simulink model "six"  (R2016b)
settings: Solver=ode4  StartTime=0.0  StopTime=10  FixedStep=0.001  RelTol=1e-3
values from neighbouring files (symbols this model uses):
  g = 9.8    [initialization.m]
  Jx = 0.007    [initialization.m]
  Jy = 0.184    [initialization.m]
  Jz = 0.184    [initialization.m]
  ksi_a = 0.6    [initialization.m]
  ksi_g = 0.7    [initialization.m]
  L = 0.9    [initialization.m]
  m = 4.81    [initialization.m]
  psiv0 = 0    [initialization.m]
  S = 0.0133    [initialization.m]
  Somega = 6*naturefrequency    [initialization.m]
  T = 1/a34    (= 0.0335307174903)    [initialization.m]
  Ta = 0.0059    [initialization.m]
  Tg = 0.006    [initialization.m]
  V0 = 1000    [initialization.m]
  xm0 = 0    [initialization.m]
  ym0 = 0    [initialization.m]
  zm0 = 0    [initialization.m]
libraries: aerolibatmos2 x1, simulink x1
settings Model: Creator=WangXuanLing  LastModifiedBy=asus
settings DataIOCC: LimitDataPoints=on  SaveFormat=Array
settings OptimizationCC: BlockReduction=off  BooleanDataType=off  LifeSpan=inf
settings DebuggingCC: SaveWithParameterizedLinksMsg=none  UnderspecifiedInitializationDetection=Classic  MergeDetectMultiDrivingBlocksExec=none  SignalResolutionControl=TryResolveAllWithWarning  SFUnexpectedBacktrackingDiag=warning  SFNoUnconditionalDefaultTransitionDiag=warning  SFExecutionAtInitializationDiag=none
settings HardwareCC: ProdBitPerPointer=32  ProdBitPerSizeT=32  ProdBitPerPtrDiffT=32  ProdLargestAtomicFloat=None  ProdIntDivRoundTo=Undefined  ProdEndianess=Unspecified  ProdWordSize=32  ProdHWDeviceType=32-bit Generic  TargetUnknown=on
settings ModelReferenceCC: PropagateSignalLabelsOutOfModel=off
settings GRTTargetCC: TargetLangStandard=C89/C90 (ANSI)  GeneratePreprocessorConditionals=Disable all
settings ConfigComp: CovMetricSettings=dw  CovHtmlReporting=on  CovSaveCumulativeToWorkspaceVar=on  CovSaveSingleToWorkspaceVar=on  CovExternalEMLEnable=off  CovSFcnEnable=off

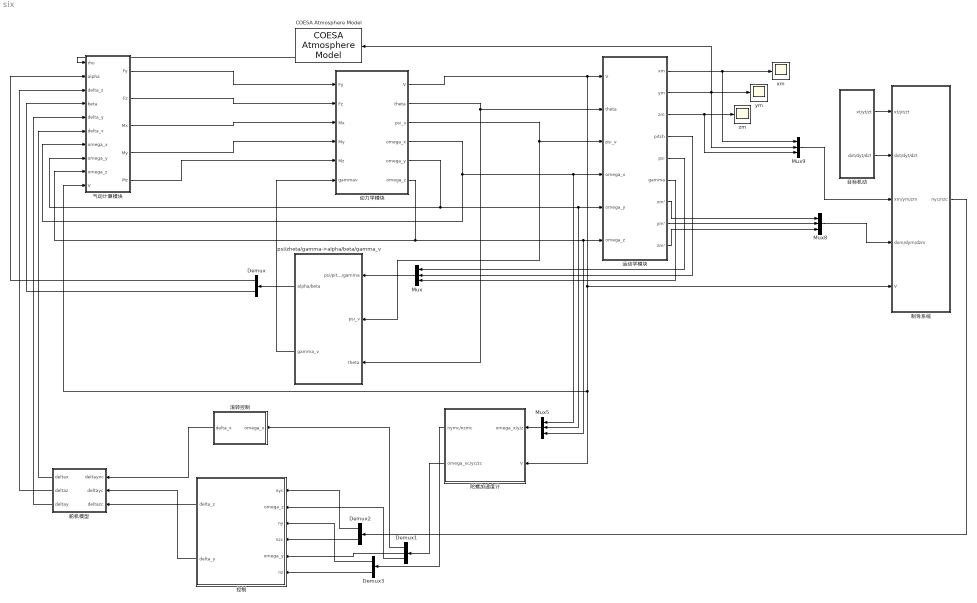
== system six ==
  COESA Atmosphere Model : aerolibatmos2/COESA Atmosphere Model  units=Metric (MKS)  spec=1976 COESA-extended U.S. Standard Atmosphere  model=Profile  profile_var=High temperature  profile_percent=1%  profile_alt=5 km (16404 ft)  envelope_var=High temperature  envelope_percent=1%  action=Warning
  Demux : Demux  Outputs=2
  Demux1 : Demux  Outputs=3
  Demux2 : Demux  Outputs=2
  Demux3 : Demux  Outputs=2
  Mux{,5,8..9} (4 alike) : Mux  Inputs=3
  psi/zheta/gamma->alpha/beta/gamma_v : Subsystem
  xm : Scope
  ym : Scope
  zm : Scope
  制导系统 : Subsystem
  动力学模块 : Subsystem
  控制 : Subsystem
  气动计算模块 : Subsystem
  滚转控制 : Subsystem
  目标机动 : Subsystem
  舵机模型 : Subsystem
  运动学模块 : Subsystem
  陀螺加速度计 : Subsystem
  wires:
  气动计算模块/1(Fy) -> 动力学模块/1(Fy)
  气动计算模块/2(Fz) -> 动力学模块/2(Fz)
  气动计算模块/3(Mx) -> 动力学模块/3(Mx)
  气动计算模块/4(My) -> 动力学模块/4(My)
  气动计算模块/5(Mz) -> 动力学模块/5(Mz)
  psi/zheta/gamma->alpha/beta/gamma_v/2(gamma_v) -> 动力学模块/6("gammav ")
  动力学模块/2(theta) -> psi/zheta/gamma->alpha/beta/gamma_v/3(theta), 运动学模块/2(theta)
  动力学模块/5(omega_y) -> 气动计算模块/8(omega_y), Mux5/2, 运动学模块/5(omega_y)
  动力学模块/6(omega_z) -> 气动计算模块/9(omega_z), Mux5/3, 运动学模块/6(omega_z)
  动力学模块/3(psi_v) -> psi/zheta/gamma->alpha/beta/gamma_v/2(psi_v), 运动学模块/3(psi_v)
  Demux/2 -> 气动计算模块/4(beta)
  Demux/1 -> 气动计算模块/2(alpha)
  运动学模块/5(psi) -> Mux/1
  运动学模块/4(pitch) -> Mux/2
  运动学模块/7(xm') -> Mux8/1
  运动学模块/8(ym') -> Mux8/2
  运动学模块/9(zm') -> Mux8/3
  动力学模块/1(V) -> 陀螺加速度计/2(V), 气动计算模块/10(V), 制导系统/5(V), 运动学模块/1(V)
  运动学模块/2(ym) -> COESA Atmosphere Model/1, ym/1, Mux9/2
  动力学模块/4(omega_x) -> 气动计算模块/7(omega_x), Mux5/1, 运动学模块/4(omega_x)
  滚转控制/1(delta_x) -> 舵机模型/1(deltayxc)
  控制/1(delta_z) -> 舵机模型/3(deltazc)
  控制/2(delta_y) -> 舵机模型/2(deltayc)
  运动学模块/6(gamma) -> Mux/3
  运动学模块/3(zm) -> zm/1, Mux9/3
  运动学模块/1(xm) -> Mux9/1, xm/1
  舵机模型/1(deltax) -> 气动计算模块/6(delta_x)
  舵机模型/2(deltaz) -> 气动计算模块/3(delta_z)
  舵机模型/3(deltay) -> 气动计算模块/5(delta_y)
  psi/zheta/gamma->alpha/beta/gamma_v/1(alpha/beta) -> Demux/1
  Mux/1 -> psi/zheta/gamma->alpha/beta/gamma_v/1(psi/pitch/gamma)
  制导系统/1(nyc/nzc) -> Demux2/1
  目标机动/2(dxt/dyt/dzt) -> 制导系统/2(dxt/dyt/dzt)
  目标机动/1(xt/yt/zt) -> 制导系统/1(xt/yt/zt)
  Mux8/1 -> 制导系统/4(dxm/dym/dzm)
  Mux9/1 -> 制导系统/3(xm/ym/zm)
  陀螺加速度计/2(omega_xc/yc/zc) -> Demux1/1
  陀螺加速度计/1(nymc/nzmc) -> Demux3/1
  Mux5/1 -> 陀螺加速度计/1(omega_x/y/z)
  COESA Atmosphere Model/4 -> 气动计算模块/1(rho)
  Demux1/1 -> 滚转控制/1(omega_x)
  Demux1/2 -> 控制/5(omega_y)
  Demux1/3 -> 控制/2(omega_z)
  Demux2/1 -> 控制/1(nyc)
  Demux2/2 -> 控制/4(nzc)
  Demux3/1 -> 控制/3(ny)
  Demux3/2 -> 控制/6(nz)

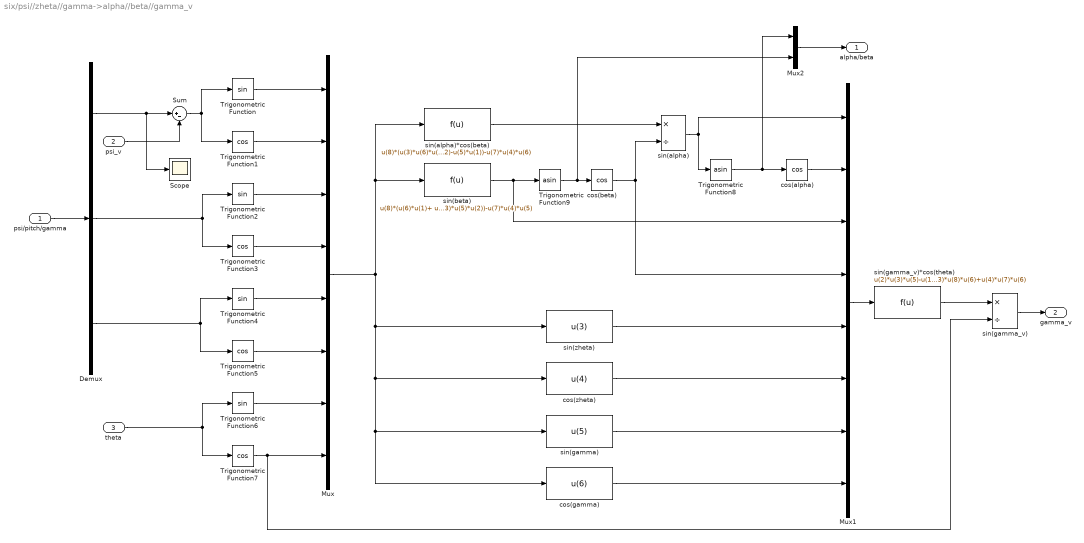
== system six/psi//zheta//gamma->alpha//beta//gamma_v ==
  psi/pitch/gamma : Inport
  psi_v : Inport  Port=2
  theta : Inport  Port=3
  Demux : Demux  Outputs=3
  Mux : Mux  Inputs=8
  Mux1 : Mux  Inputs=8
  Mux2 : Mux  Inputs=2
  Scope : Scope
  Sum : Sum  Inputs=|+-
  Trigonometric Function{,2,4,6} (4 alike) : Trigonometry
  Trigonometric Function{1,3,5,7} (4 alike) : Trigonometry  Operator=cos
  Trigonometric Function8 : Trigonometry  Operator=asin
  Trigonometric Function9 : Trigonometry  Operator=asin
  cos(alpha) : Trigonometry  Operator=cos
  cos(beta) : Trigonometry  Operator=cos
  cos(gamma) : Fcn  Expr=u(6)
  cos(zheta) : Fcn  Expr=u(4)
  sin(alpha) : Product  Inputs=*/
  sin(alpha)*cos(beta) : Fcn  Expr=u(8)*(u(3)*u(6)*u(2)-u(5)*u(1))-u(7)*u(4)*u(6)
  sin(beta) : Fcn  Expr=u(8)*(u(6)*u(1)+ u(3)*u(5)*u(2))-u(7)*u(4)*u(5)
  sin(gamma) : Fcn  Expr=u(5)
  sin(gamma_v) : Product  Inputs=*/
  sin(gamma_v)*cos(theta) : Fcn  Expr=u(2)*u(3)*u(5)-u(1)*u(3)*u(8)*u(6)+u(4)*u(7)*u(6)
  sin(zheta) : Fcn  Expr=u(3)
  alpha/beta : Outport
  gamma_v : Outport  Port=2
  wires:
  psi/pitch/gamma/1 -> Demux/1
  Demux/1 -> Scope/1, Sum/1
  Sum/1 -> Trigonometric Function/1, Trigonometric Function1/1
  Demux/2 -> Trigonometric Function3/1, Trigonometric Function2/1
  Demux/3 -> Trigonometric Function4/1, Trigonometric Function5/1
  Trigonometric Function/1 -> Mux/1
  Trigonometric Function1/1 -> Mux/2
  Trigonometric Function2/1 -> Mux/3
  Trigonometric Function3/1 -> Mux/4
  Trigonometric Function4/1 -> Mux/5
  Trigonometric Function5/1 -> Mux/6
  theta/1 -> Trigonometric Function7/1, Trigonometric Function6/1
  Trigonometric Function6/1 -> Mux/7
  Trigonometric Function7/1 -> Mux/8, sin(gamma_v)/2
  sin(beta)/1 -> Mux1/3, Trigonometric Function9/1
  Trigonometric Function9/1 -> Mux2/2, cos(beta)/1
  sin(alpha)*cos(beta)/1 -> sin(alpha)/1
  cos(beta)/1 -> Mux1/4, sin(alpha)/2
  sin(alpha)/1 -> Mux1/1, Trigonometric Function8/1
  Trigonometric Function8/1 -> Mux2/1, cos(alpha)/1
  cos(alpha)/1 -> Mux1/2
  sin(zheta)/1 -> Mux1/5
  cos(zheta)/1 -> Mux1/6
  sin(gamma)/1 -> Mux1/7
  cos(gamma)/1 -> Mux1/8
  sin(gamma_v)*cos(theta)/1 -> sin(gamma_v)/1
  sin(gamma_v)/1 -> gamma_v/1
  psi_v/1 -> Sum/2
  Mux/1 -> cos(gamma)/1, sin(gamma)/1, cos(zheta)/1, sin(zheta)/1, sin(alpha)*cos(beta)/1, sin(beta)/1
  Mux1/1 -> sin(gamma_v)*cos(theta)/1
  Mux2/1 -> alpha/beta/1

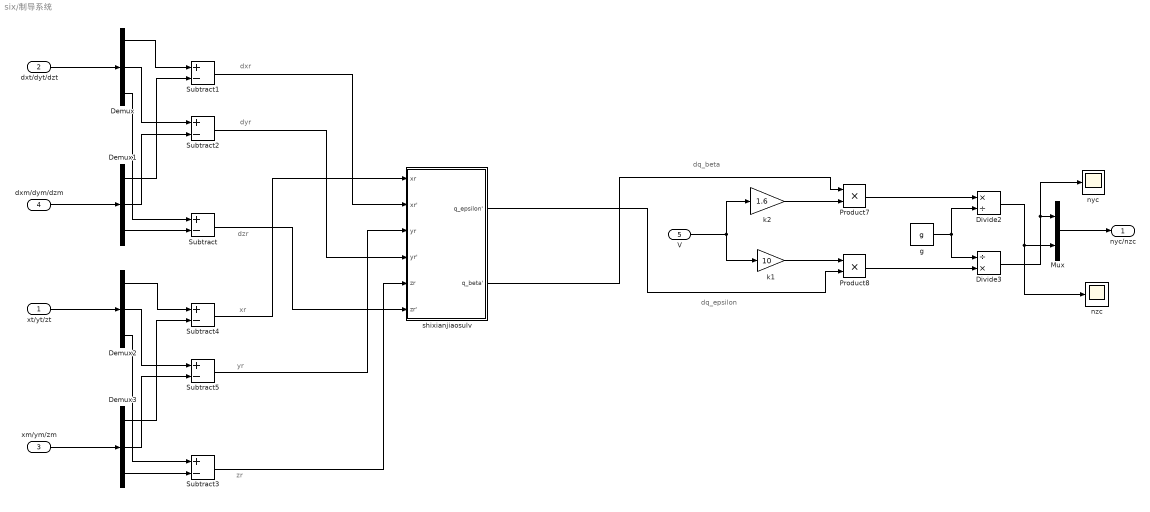
== system six/制导系统 ==
  note: dq_epsilon
  note: zr
  note: yr
  note: xr
  note: dzr
  note: dyr
  note: dxr
  note: dq_beta
  xt/yt/zt : Inport
  dxt/dyt/dzt : Inport  Port=2
  xm/ym/zm : Inport  Port=3
  dxm/dym/dzm : Inport  Port=4
  V : Inport  Port=5
  Demux{,1..3} (4 alike) : Demux  Outputs=3
  Divide2 : Product  Inputs=*/
  Divide3 : Product  Inputs=/*
  Mux : Mux  Inputs=2
  Product7 : Product
  Product8 : Product
  Subtract{,1..5} (6 alike) : Sum  Inputs=+-
  g : Constant  Value=g
  k1 : Gain  Gain=10
  k2 : Gain  Gain=1.6
  nyc : Scope
  nzc : Scope
  shixianjiaosulv : Subsystem
  nyc/nzc : Outport
  wires:
  Demux/3 -> Subtract/1
  Demux/2 -> Subtract2/1
  dxm/dym/dzm/1 -> Demux1/1
  dxt/dyt/dzt/1 -> Demux/1
  k2/1 -> Product7/2
  Subtract5/1 -> shixianjiaosulv/3(yr)
  Product7/1 -> Divide2/1
  g/1 -> Divide3/1, Divide2/2
  Demux3/3 -> Subtract3/2
  Mux/1 -> nyc/nzc/1
  Demux1/3 -> Subtract/2
  Demux2/1 -> Subtract4/1
  V/1 -> k1/1, k2/1
  Demux3/1 -> Subtract4/2
  Product8/1 -> Divide3/2
  Demux2/2 -> Subtract5/1
  xm/ym/zm/1 -> Demux3/1
  xt/yt/zt/1 -> Demux2/1
  Subtract3/1 -> shixianjiaosulv/5(zr)
  k1/1 -> Product8/1
  Demux3/2 -> Subtract5/2
  Demux2/3 -> Subtract3/1
  Demux1/1 -> Subtract1/2
  Demux/1 -> Subtract1/1
  Demux1/2 -> Subtract2/2
  Divide2/1 -> nzc/1, Mux/2
  Divide3/1 -> Mux/1, nyc/1
  shixianjiaosulv/1(q_epsilon') -> Product8/2
  shixianjiaosulv/2(q_beta') -> Product7/1
  Subtract4/1 -> shixianjiaosulv/1(xr)
  Subtract1/1 -> shixianjiaosulv/2(xr')
  Subtract2/1 -> shixianjiaosulv/4(yr')
  Subtract/1 -> shixianjiaosulv/6(zr')

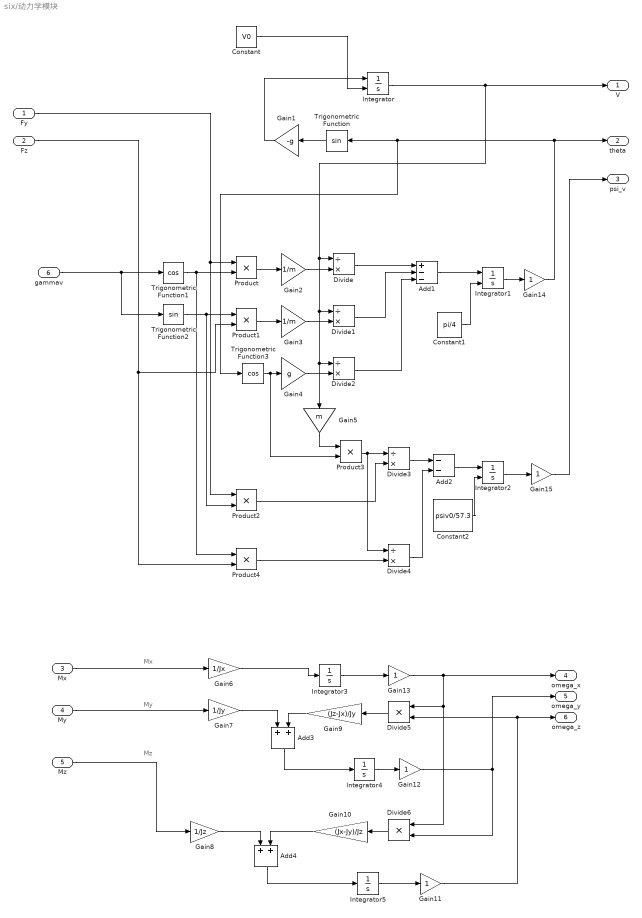
== system six/动力学模块 ==
  note: Mz
  note: My
  note: Mx
  Fy : Inport
  Fz : Inport  Port=2
  Mx : Inport  Port=3
  My : Inport  Port=4
  Mz : Inport  Port=5
  "gammav " : Inport  Port=6
  Add1 : Sum  Inputs=+--
  Add2 : Sum  Inputs=--
  Add3 : Sum
  Add4 : Sum
  Constant : Constant  Value=V0
  Constant1 : Constant  Value=pi/4
  Constant2 : Constant  Value=psiv0/57.3
  Divide{,1..4} (5 alike) : Product  Inputs=/*
  Divide5 : Product  Inputs=**
  Divide6 : Product  Inputs=**
  Gain1 : Gain  Gain=-g
  Gain10 : Gain  Gain=(Jx-Jy)/Jz
  Gain{11..15} (5 alike) : Gain
  Gain2 : Gain  Gain=1/m
  Gain3 : Gain  Gain=1/m
  Gain4 : Gain  Gain=g
  Gain5 : Gain  Gain=m
  Gain6 : Gain  Gain=1/Jx
  Gain7 : Gain  Gain=1/Jy
  Gain8 : Gain  Gain=1/Jz
  Gain9 : Gain  Gain=(Jz-Jx)/Jy
  Integrator : Integrator  InitialConditionSource=external
  Integrator1 : Integrator  InitialConditionSource=external
  Integrator2 : Integrator  InitialConditionSource=external
  Integrator3 : Integrator
  Integrator4 : Integrator
  Integrator5 : Integrator
  Product{,1..4} (5 alike) : Product
  Trigonometric Function : Trigonometry
  Trigonometric Function1 : Trigonometry  Operator=cos
  Trigonometric Function2 : Trigonometry
  Trigonometric Function3 : Trigonometry  Operator=cos
  V : Outport
  theta : Outport  Port=2
  psi_v : Outport  Port=3
  omega_x : Outport  Port=4
  omega_y : Outport  Port=5
  omega_z : Outport  Port=6
  wires:
  Fy/1 -> Product/1, Product2/1
  Fz/1 -> Product4/2, Product1/2
  Trigonometric Function/1 -> Gain1/1
  Gain1/1 -> Integrator/1
  "gammav "/1 -> Trigonometric Function2/1, Trigonometric Function1/1
  Trigonometric Function1/1 -> Product4/1, Product/2
  Product/1 -> Gain2/1
  Gain2/1 -> Divide/2
  Gain3/1 -> Divide1/2
  Product1/1 -> Gain3/1
  Divide/1 -> Add1/1
  Divide1/1 -> Add1/2
  Constant/1 -> Integrator/2
  Trigonometric Function3/1 -> Product3/2, Gain4/1
  Gain4/1 -> Divide2/2
  Divide2/1 -> Add1/3
  Add1/1 -> Integrator1/1
  Constant1/1 -> Integrator1/2
  Trigonometric Function2/1 -> Product1/1, Product2/2
  Gain5/1 -> Product3/1
  Product3/1 -> Divide4/1, Divide3/1
  Product2/1 -> Divide3/2
  Divide3/1 -> Add2/1
  Product4/1 -> Divide4/2
  Divide4/1 -> Add2/2
  Add2/1 -> Integrator2/1
  Constant2/1 -> Integrator2/2
  Mx/1 -> Gain6/1
  My/1 -> Gain7/1
  Mz/1 -> Gain8/1
  Gain6/1 -> Integrator3/1
  Integrator3/1 -> Gain13/1
  Gain7/1 -> Add3/1
  Divide5/1 -> Gain9/1
  Gain9/1 -> Add3/2
  Add3/1 -> Integrator4/1
  Gain8/1 -> Add4/1
  Gain12/1 -> omega_y/1, Divide6/2
  Divide6/1 -> Gain10/1
  Gain10/1 -> Add4/2
  Add4/1 -> Integrator5/1
  Gain11/1 -> Divide5/2, omega_z/1
  Integrator/1 -> V/1, Divide/1, Gain5/1, Divide2/1, Divide1/1
  Integrator1/1 -> Gain14/1
  Integrator2/1 -> Gain15/1
  Integrator5/1 -> Gain11/1
  Integrator4/1 -> Gain12/1
  Gain14/1 -> theta/1, Trigonometric Function/1, Trigonometric Function3/1
  Gain15/1 -> psi_v/1
  Gain13/1 -> omega_x/1, Divide6/1, Divide5/1

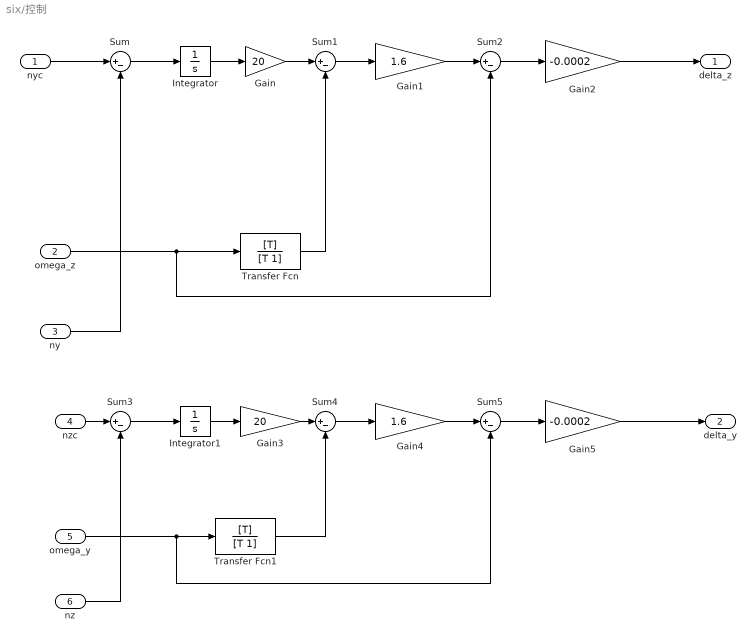
== system six/控制 ==
  nyc : Inport
  omega_z : Inport  Port=2
  ny : Inport  Port=3
  nzc : Inport  Port=4
  omega_y : Inport  Port=5
  nz : Inport  Port=6
  Gain : Gain  Gain=20
  Gain1 : Gain  Gain=1.6
  Gain2 : Gain  Gain=-0.0002
  Gain3 : Gain  Gain=20
  Gain4 : Gain  Gain=1.6
  Gain5 : Gain  Gain=-0.0002
  Integrator : Integrator
  Integrator1 : Integrator
  Sum{,1..5} (6 alike) : Sum  Inputs=|+-
  Transfer Fcn : TransferFcn  Numerator=[T]  Denominator=[T 1]
  Transfer Fcn1 : TransferFcn  Numerator=[T]  Denominator=[T 1]
  delta_z : Outport
  delta_y : Outport  Port=2
  wires:
  Sum3/1 -> Integrator1/1
  Integrator/1 -> Gain/1
  Sum4/1 -> Gain4/1
  Sum/1 -> Integrator/1
  Integrator1/1 -> Gain3/1
  Sum2/1 -> Gain2/1
  Gain4/1 -> Sum5/1
  Sum1/1 -> Gain1/1
  Gain1/1 -> Sum2/1
  Sum5/1 -> Gain5/1
  Gain3/1 -> Sum4/1
  Gain/1 -> Sum1/1
  Gain2/1 -> delta_z/1
  Gain5/1 -> delta_y/1
  omega_y/1 -> Sum5/2, Transfer Fcn1/1
  Transfer Fcn1/1 -> Sum4/2
  nyc/1 -> Sum/1
  ny/1 -> Sum/2
  omega_z/1 -> Sum2/2, Transfer Fcn/1
  Transfer Fcn/1 -> Sum1/2
  nz/1 -> Sum3/2
  nzc/1 -> Sum3/1

== system six/气动计算模块 ==
  rho : Inport
  alpha : Inport  Port=2
  delta_z : Inport  Port=3
  beta : Inport  Port=4
  delta_y : Inport  Port=5
  delta_x : Inport  Port=6
  omega_x : Inport  Port=7
  omega_y : Inport  Port=8
  omega_z : Inport  Port=9
  V : Inport  Port=10
  Gain : Gain  Gain=0.5
  Product : Product  Inputs=3
  qidongli : Subsystem
  qidongliju : Subsystem
  Fy : Outport
  Fz : Outport  Port=2
  Mx : Outport  Port=3
  My : Outport  Port=4
  Mz : Outport  Port=5
  wires:
  qidongli/2(Fz) -> Fz/1
  delta_x/1 -> qidongliju/1(delta_x)
  delta_y/1 -> qidongliju/4(delta_y), qidongli/5(delta_y)
  beta/1 -> qidongli/4(beta), qidongliju/6(beta)
  delta_z/1 -> qidongli/2(delta_z), qidongliju/7(delta_z)
  Gain/1 -> qidongli/3(q), qidongliju/3(q)
  alpha/1 -> qidongli/1(alpha), qidongliju/9(alpha)
  qidongliju/1(Mx) -> Mx/1
  qidongliju/2(My) -> My/1
  qidongli/1(Fy) -> Fy/1
  V/1 -> Product/1, Product/2
  Product/1 -> Gain/1
  rho/1 -> Product/3
  omega_x/1 -> qidongliju/2(omega_x)
  omega_y/1 -> qidongliju/5(omega_y)
  omega_z/1 -> qidongliju/8(omega_z)
  qidongliju/3(Mz) -> Mz/1

== system six/滚转控制 ==
  omega_x : Inport
  Integrator : Integrator
  Ka1 : Gain  Gain=70
  Ka2 : Gain  Gain=0
  Kb1 : Gain  Gain=-0.015
  Sine Wave : Sin  Amplitude=1/57.3  Frequency=10  SampleTime=0
  Sum2 : Sum  Inputs=|+-
  Sum3 : Sum  Inputs=|+-
  delta_x : Outport
  wires:
  Sine Wave/1 -> Ka2/1
  Sum2/1 -> Ka1/1
  Sum3/1 -> Kb1/1
  Kb1/1 -> delta_x/1
  omega_x/1 -> Integrator/1, Sum3/2
  Ka2/1 -> Sum2/1
  Ka1/1 -> Sum3/1
  Integrator/1 -> Sum2/2

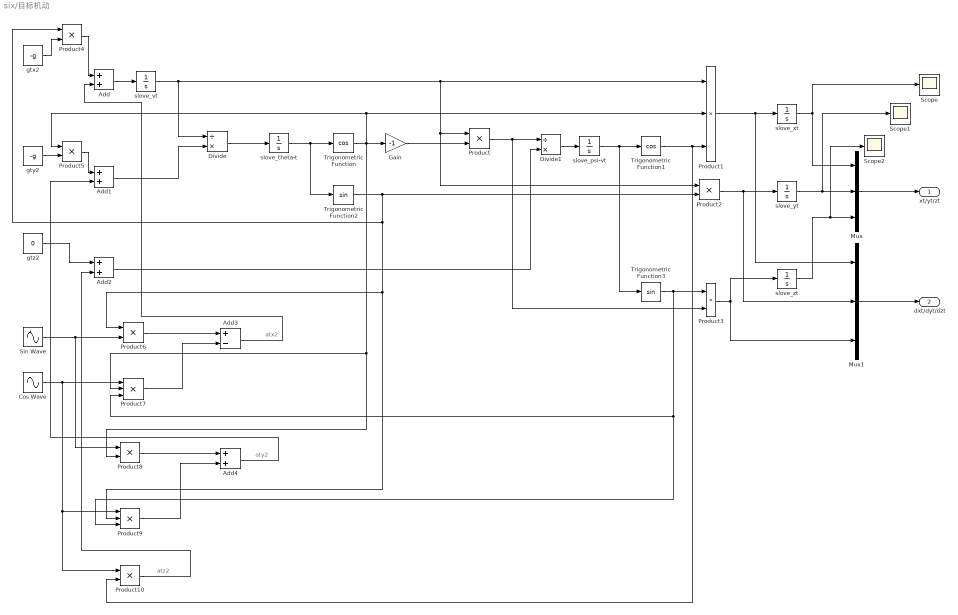
== system six/目标机动 ==
  note: atz2
  note: aty2
  note: atx2
  Add{,1..2,4} (4 alike) : Sum
  Add3 : Sum  Inputs=+-
  Cos Wave : Sin  Amplitude=7*9.8  Phase=pi/2  SampleTime=0
  Divide : Product  Inputs=/*
  Divide1 : Product  Inputs=/*
  Gain : Gain  Gain=-1
  Mux : Mux  Inputs=3
  Mux1 : Mux  Inputs=3
  Product{,2..6,8,10} (8 alike) : Product
  Product1 : Product  Inputs=3
  Product7 : Product  Inputs=3
  Product9 : Product  Inputs=3
  Scope : Scope
  Scope1 : Scope
  Scope2 : Scope
  Sin Wave : Sin  Amplitude=7*9.8  SampleTime=0
  Trigonometric Function : Trigonometry  Operator=cos
  Trigonometric Function1 : Trigonometry  Operator=cos
  Trigonometric Function2 : Trigonometry
  Trigonometric Function3 : Trigonometry
  gtx2 : Constant  Value=-g
  gty2 : Constant  Value=-g
  gtz2 : Constant  Value=0
  slove_psi-vt : Integrator  InitialCondition=120/57.3
  slove_theta-t : Integrator  InitialCondition=-30/57.3
  slove_vt : Integrator  InitialCondition=800
  slove_xt : Integrator  InitialCondition=11136
  slove_yt : Integrator  InitialCondition=8603.6
  slove_zt : Integrator  InitialCondition=5192.8
  xt/yt/zt : Outport
  dxt/dyt/dzt : Outport  Port=2
  wires:
  Trigonometric Function2/1 -> Product9/2, Product6/1, Product4/1, Product2/2
  Product2/1 -> Mux1/2, slove_yt/1
  Trigonometric Function3/1 -> Product9/3, Product7/3, Product3/1
  Trigonometric Function1/1 -> Product10/2, Product1/3
  Product3/1 -> Mux1/3, slove_zt/1
  Mux/1 -> xt/yt/zt/1
  Product1/1 -> Mux1/1, slove_xt/1
  gtz2/1 -> Add2/1
  Add2/1 -> Divide1/2
  Divide/1 -> slove_theta-t/1
  slove_zt/1 -> Scope2/1, Mux/3
  Product/1 -> Product3/2, Divide1/1
  slove_vt/1 -> Product2/1, Product/1, Product1/1, Divide/1
  slove_theta-t/1 -> Trigonometric Function2/1, Trigonometric Function/1
  Add/1 -> slove_vt/1
  Add1/1 -> Divide/2
  slove_xt/1 -> Scope/1, Mux/1
  Trigonometric Function/1 -> Product8/2, Product7/2, Product5/1, Product1/2, Gain/1
  Divide1/1 -> slove_psi-vt/1
  Gain/1 -> Product/2
  slove_psi-vt/1 -> Trigonometric Function3/1, Trigonometric Function1/1
  slove_yt/1 -> Scope1/1, Mux/2
  Mux1/1 -> dxt/dyt/dzt/1
  gtx2/1 -> Product4/2
  Product4/1 -> Add/1
  gty2/1 -> Product5/2
  Product5/1 -> Add1/1
  Product10/1 -> Add2/2
  Add4/1 -> Add1/2
  Sin Wave/1 -> Product8/1, Product6/2
  Cos Wave/1 -> Product10/1, Product9/1, Product7/1
  Product6/1 -> Add3/1
  Product7/1 -> Add3/2
  Add3/1 -> Add/2
  Product8/1 -> Add4/1
  Product9/1 -> Add4/2

== system six/舵机模型 ==
  deltayxc : Inport
  deltayc : Inport  Port=2
  deltazc : Inport  Port=3
  Transfer Fcn : TransferFcn  Numerator=[Somega*Somega]  Denominator=[1 1.4*Somega Somega*Somega]
  Transfer Fcn1 : TransferFcn  Numerator=[Somega*Somega]  Denominator=[1 1.4*Somega Somega*Somega]
  滚转舵机 : TransferFcn  Numerator=[Somega*Somega]  Denominator=[1 1.4*Somega Somega*Somega]
  deltax : Outport
  deltaz : Outport  Port=2
  deltay : Outport  Port=3
  wires:
  deltazc/1 -> Transfer Fcn/1
  Transfer Fcn/1 -> deltaz/1
  deltayc/1 -> Transfer Fcn1/1
  Transfer Fcn1/1 -> deltay/1
  deltayxc/1 -> 滚转舵机/1
  滚转舵机/1 -> deltax/1

== system six/运动学模块 ==
  V : Inport
  theta : Inport  Port=2
  psi_v : Inport  Port=3
  omega_x : Inport  Port=4
  omega_y : Inport  Port=5
  omega_z : Inport  Port=6
  juli : Subsystem
  zhuandongjiaodu : Subsystem
  xm : Outport
  ym : Outport  Port=2
  zm : Outport  Port=3
  pitch : Outport  Port=4
  psi : Outport  Port=5
  gamma : Outport  Port=6
  xm' : Outport  Port=7
  ym' : Outport  Port=8
  zm' : Outport  Port=9
  wires:
  zhuandongjiaodu/3(gamma) -> gamma/1
  omega_x/1 -> zhuandongjiaodu/1(omega_x)
  omega_y/1 -> zhuandongjiaodu/2(omega_y)
  omega_z/1 -> zhuandongjiaodu/3(omega_z)
  zhuandongjiaodu/1(pitch) -> pitch/1
  zhuandongjiaodu/2(psi) -> psi/1
  juli/1(xm) -> xm/1
  psi_v/1 -> juli/3(psi_v)
  theta/1 -> juli/2(theta)
  juli/2(ym) -> ym/1
  juli/3(zm) -> zm/1
  V/1 -> juli/1(V)
  juli/5(ym') -> ym'/1
  juli/6(zm') -> zm'/1
  juli/4(xm') -> xm'/1

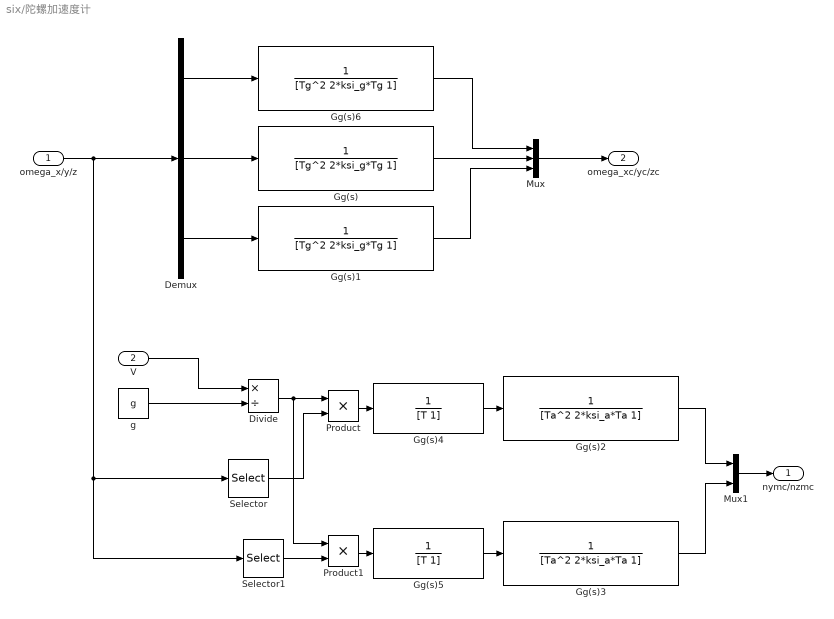
== system six/陀螺加速度计 ==
  omega_x/y/z : Inport
  V : Inport  Port=2
  " Gg(s)" : TransferFcn  Denominator=[Tg^2 2*ksi_g*Tg 1]
  " Gg(s)1" : TransferFcn  Denominator=[Tg^2 2*ksi_g*Tg 1]
  " Gg(s)2" : TransferFcn  Denominator=[Ta^2 2*ksi_a*Ta 1]
  " Gg(s)3" : TransferFcn  Denominator=[Ta^2 2*ksi_a*Ta 1]
  " Gg(s)4" : TransferFcn  Denominator=[T 1]
  " Gg(s)5" : TransferFcn  Denominator=[T 1]
  " Gg(s)6" : TransferFcn  Denominator=[Tg^2 2*ksi_g*Tg 1]
  Demux : Demux  Outputs=3
  Divide : Product  Inputs=*/
  Mux : Mux  Inputs=3
  Mux1 : Mux  Inputs=2
  Product : Product
  Product1 : Product
  Selector : Selector  InputPortWidth=3  IndexOptions=Index vector (dialog)  Indices=3  OutputSizes=1
  Selector1 : Selector  InputPortWidth=3  IndexOptions=Index vector (dialog)  Indices=2  OutputSizes=1
  g : Constant  Value=g
  nymc/nzmc : Outport
  omega_xc/yc/zc : Outport  Port=2
  wires:
  omega_x/y/z/1 -> Selector1/1, Selector/1, Demux/1
  Demux/2 -> " Gg(s)"/1
  Demux/3 -> " Gg(s)1"/1
  Mux/1 -> omega_xc/yc/zc/1
  V/1 -> Divide/1
  g/1 -> Divide/2
  " Gg(s)4"/1 -> " Gg(s)2"/1
  " Gg(s)5"/1 -> " Gg(s)3"/1
  Divide/1 -> Product/1, Product1/1
  Selector/1 -> Product/2
  Product/1 -> " Gg(s)4"/1
  Selector1/1 -> Product1/2
  Product1/1 -> " Gg(s)5"/1
  " Gg(s)2"/1 -> Mux1/1
  " Gg(s)3"/1 -> Mux1/2
  Mux1/1 -> nymc/nzmc/1
  Demux/1 -> " Gg(s)6"/1
  " Gg(s)1"/1 -> Mux/3
  " Gg(s)"/1 -> Mux/2
  " Gg(s)6"/1 -> Mux/1

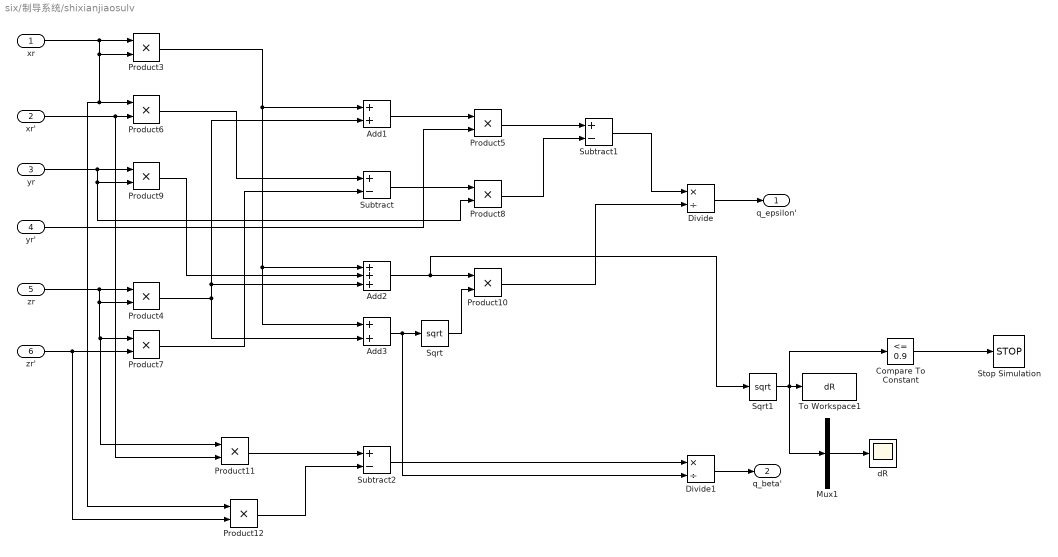
== system six/制导系统/shixianjiaosulv ==
  xr : Inport
  xr' : Inport  Port=2
  yr : Inport  Port=3
  yr' : Inport  Port=4
  zr : Inport  Port=5
  zr' : Inport  Port=6
  Add1 : Sum
  Add2 : Sum  Inputs=+++
  Add3 : Sum
  Compare To Constant : simulink/Logic and Bit Operations/Compare To Constant  relop=<=  const=0.9  OutDataTypeStr=boolean
  Divide : Product  Inputs=*/
  Divide1 : Product  Inputs=*/
  Mux1 : Mux  Inputs=1
  Product{3..12} (10 alike) : Product
  Sqrt : Sqrt  SaturateOnIntegerOverflow=on
  Sqrt1 : Sqrt  SaturateOnIntegerOverflow=on
  Stop Simulation : Stop
  Subtract : Sum  Inputs=+-
  Subtract1 : Sum  Inputs=+-
  Subtract2 : Sum  Inputs=+-
  To Workspace1 : ToWorkspace  VariableName=dR  SaveFormat=Timeseries  SampleTime=-1
  dR : Scope
  q_epsilon' : Outport
  q_beta' : Outport  Port=2
  wires:
  Product6/1 -> Subtract/1
  Divide/1 -> q_epsilon'/1
  Subtract2/1 -> Divide1/1
  Add1/1 -> Product5/1
  yr'/1 -> Product5/2
  Product12/1 -> Subtract2/2
  Subtract/1 -> Product8/1
  Product8/1 -> Subtract1/2
  zr'/1 -> Product12/2, Product7/2
  Subtract1/1 -> Divide/1
  xr/1 -> Product6/1, Product12/1, Product3/2, Product3/1
  yr/1 -> Product9/1, Product8/2, Product9/2
  Product3/1 -> Add1/1, Add2/1, Add3/1
  Product10/1 -> Divide/2
  Product4/1 -> Add3/2, Add2/3, Add1/2
  Divide1/1 -> q_beta'/1
  xr'/1 -> Product11/2, Product6/2
  Product7/1 -> Subtract/2
  Sqrt/1 -> Product10/2
  zr/1 -> Product11/1, Product7/1, Product4/2, Product4/1
  Product9/1 -> Add2/2
  Product11/1 -> Subtract2/1
  Product5/1 -> Subtract1/1
  Add3/1 -> Divide1/2, Sqrt/1
  Add2/1 -> Sqrt1/1, Product10/1
  Sqrt1/1 -> Compare To Constant/1, Mux1/1, To Workspace1/1
  Mux1/1 -> dR/1
  Compare To Constant/1 -> Stop Simulation/1

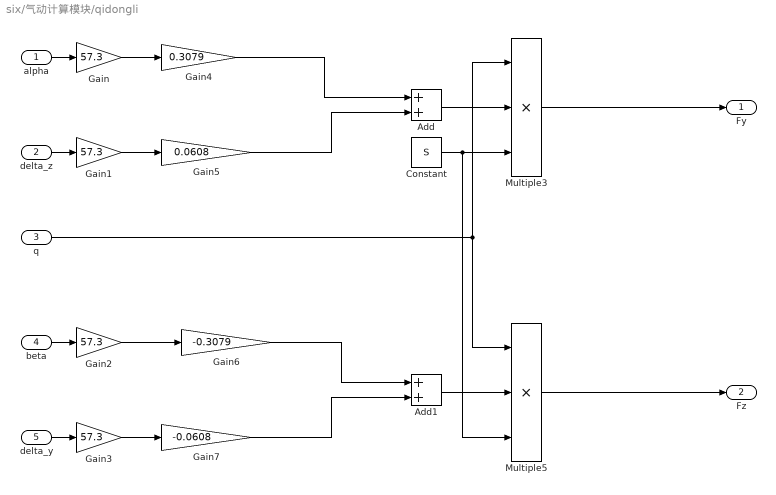
== system six/气动计算模块/qidongli ==
  alpha : Inport
  delta_z : Inport  Port=2
  q : Inport  Port=3
  beta : Inport  Port=4
  delta_y : Inport  Port=5
  Add : Sum
  Add1 : Sum
  Constant : Constant  Value=S
  Gain{,1..3} (4 alike) : Gain  Gain=57.3
  Gain4 : Gain  Gain=0.3079
  Gain5 : Gain  Gain=0.0608
  Gain6 : Gain  Gain=-0.3079
  Gain7 : Gain  Gain=-0.0608
  Multiple3 : Product  Inputs=***
  Multiple5 : Product  Inputs=***
  Fy : Outport
  Fz : Outport  Port=2
  wires:
  Add1/1 -> Multiple5/2
  q/1 -> Multiple3/1, Multiple5/1
  Constant/1 -> Multiple5/3, Multiple3/3
  Multiple5/1 -> Fz/1
  Multiple3/1 -> Fy/1
  Add/1 -> Multiple3/2
  alpha/1 -> Gain/1
  Gain/1 -> Gain4/1
  Gain1/1 -> Gain5/1
  delta_z/1 -> Gain1/1
  Gain2/1 -> Gain6/1
  beta/1 -> Gain2/1
  Gain3/1 -> Gain7/1
  delta_y/1 -> Gain3/1
  Gain4/1 -> Add/1
  Gain5/1 -> Add/2
  Gain6/1 -> Add1/1
  Gain7/1 -> Add1/2

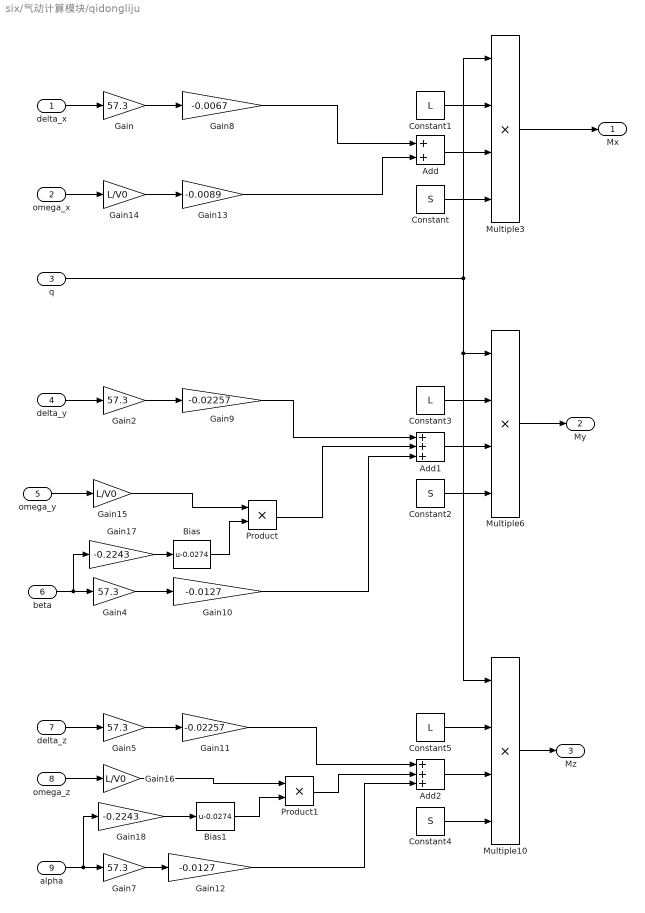
== system six/气动计算模块/qidongliju ==
  delta_x : Inport
  omega_x : Inport  Port=2
  q : Inport  Port=3
  delta_y : Inport  Port=4
  omega_y : Inport  Port=5
  beta : Inport  Port=6
  delta_z : Inport  Port=7
  omega_z : Inport  Port=8
  alpha : Inport  Port=9
  Add : Sum
  Add1 : Sum  Inputs=+++
  Add2 : Sum  Inputs=+++
  Bias : Bias  Bias=-0.0274
  Bias1 : Bias  Bias=-0.0274
  Constant : Constant  Value=S
  Constant1 : Constant  Value=L
  Constant2 : Constant  Value=S
  Constant3 : Constant  Value=L
  Constant4 : Constant  Value=S
  Constant5 : Constant  Value=L
  Gain{,2,4..5,7} (5 alike) : Gain  Gain=57.3
  Gain10 : Gain  Gain=-0.0127
  Gain11 : Gain  Gain=-0.02257
  Gain12 : Gain  Gain=-0.0127
  Gain13 : Gain  Gain=-0.0089
  Gain14 : Gain  Gain=L/V0
  Gain15 : Gain  Gain=L/V0
  Gain16 : Gain  Gain=L/V0
  Gain17 : Gain  Gain=-0.2243
  Gain18 : Gain  Gain=-0.2243
  Gain8 : Gain  Gain=-0.0067
  Gain9 : Gain  Gain=-0.02257
  Multiple10 : Product  Inputs=****
  Multiple3 : Product  Inputs=****
  Multiple6 : Product  Inputs=****
  Product : Product
  Product1 : Product
  Mx : Outport
  My : Outport  Port=2
  Mz : Outport  Port=3
  wires:
  Constant1/1 -> Multiple3/2
  Constant/1 -> Multiple3/4
  q/1 -> Multiple3/1, Multiple10/1, Multiple6/1
  Multiple6/1 -> My/1
  omega_x/1 -> Gain14/1
  delta_x/1 -> Gain/1
  omega_z/1 -> Gain16/1
  Gain/1 -> Gain8/1
  Gain7/1 -> Gain12/1
  delta_z/1 -> Gain5/1
  beta/1 -> Gain17/1, Gain4/1
  Gain4/1 -> Gain10/1
  Gain2/1 -> Gain9/1
  alpha/1 -> Gain18/1, Gain7/1
  delta_y/1 -> Gain2/1
  Multiple10/1 -> Mz/1
  Add1/1 -> Multiple6/3
  Constant2/1 -> Multiple6/4
  Constant3/1 -> Multiple6/2
  omega_y/1 -> Gain15/1
  Add/1 -> Multiple3/3
  Gain10/1 -> Add1/3
  Constant4/1 -> Multiple10/4
  Add2/1 -> Multiple10/3
  Constant5/1 -> Multiple10/2
  Gain14/1 -> Gain13/1
  Gain13/1 -> Add/2
  Gain8/1 -> Add/1
  Gain9/1 -> Add1/1
  Gain11/1 -> Add2/1
  Gain5/1 -> Gain11/1
  Gain12/1 -> Add2/3
  Multiple3/1 -> Mx/1
  Product/1 -> Add1/2
  Gain15/1 -> Product/1
  Product1/1 -> Add2/2
  Gain16/1 -> Product1/1
  Gain17/1 -> Bias/1
  Bias/1 -> Product/2
  Gain18/1 -> Bias1/1
  Bias1/1 -> Product1/2

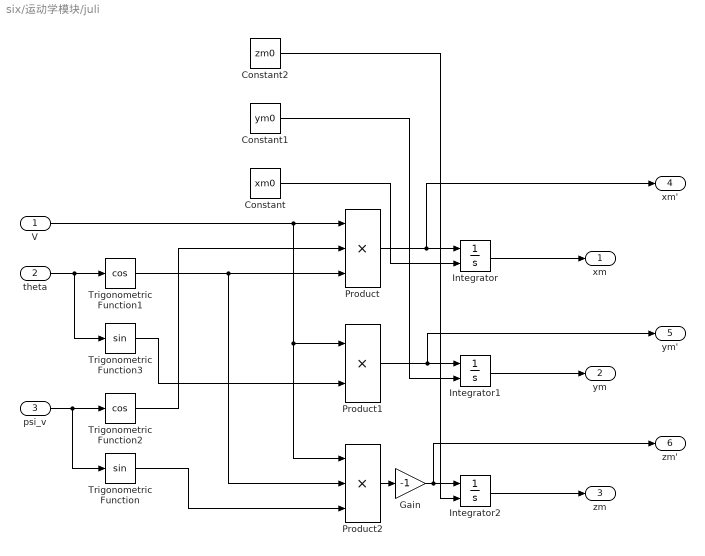
== system six/运动学模块/juli ==
  V : Inport
  theta : Inport  Port=2
  psi_v : Inport  Port=3
  Constant : Constant  Value=xm0
  Constant1 : Constant  Value=ym0
  Constant2 : Constant  Value=zm0
  Gain : Gain  Gain=-1
  Integrator : Integrator  InitialConditionSource=external
  Integrator1 : Integrator  InitialConditionSource=external
  Integrator2 : Integrator  InitialConditionSource=external
  Product : Product  Inputs=3
  Product1 : Product
  Product2 : Product  Inputs=3
  Trigonometric Function : Trigonometry
  Trigonometric Function1 : Trigonometry  Operator=cos
  Trigonometric Function2 : Trigonometry  Operator=cos
  Trigonometric Function3 : Trigonometry
  xm : Outport
  ym : Outport  Port=2
  zm : Outport  Port=3
  xm' : Outport  Port=4
  ym' : Outport  Port=5
  zm' : Outport  Port=6
  wires:
  V/1 -> Product2/1, Product1/1, Product/1
  Integrator1/1 -> ym/1
  Constant/1 -> Integrator/2
  Integrator/1 -> xm/1
  Trigonometric Function3/1 -> Product1/2
  psi_v/1 -> Trigonometric Function/1, Trigonometric Function2/1
  Product1/1 -> ym'/1, Integrator1/1
  Trigonometric Function1/1 -> Product2/2, Product/3
  Trigonometric Function/1 -> Product2/3
  Gain/1 -> zm'/1, Integrator2/1
  Integrator2/1 -> zm/1
  Product2/1 -> Gain/1
  Product/1 -> xm'/1, Integrator/1
  Constant2/1 -> Integrator2/2
  theta/1 -> Trigonometric Function3/1, Trigonometric Function1/1
  Trigonometric Function2/1 -> Product/2
  Constant1/1 -> Integrator1/2

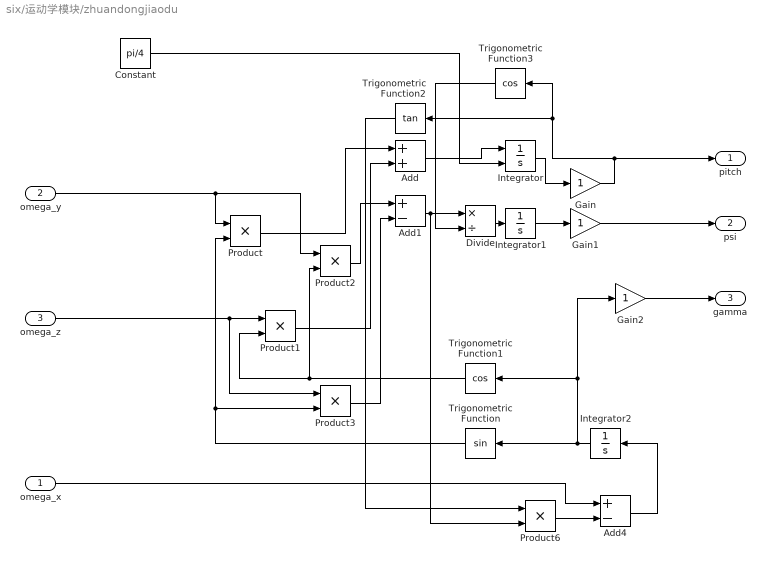
== system six/运动学模块/zhuandongjiaodu ==
  omega_x : Inport
  omega_y : Inport  Port=2
  omega_z : Inport  Port=3
  Add : Sum
  Add1 : Sum  Inputs=+-
  Add4 : Sum  Inputs=+-
  Constant : Constant  Value=pi/4
  Divide : Product  Inputs=*/
  Gain : Gain
  Gain1 : Gain
  Gain2 : Gain
  Integrator : Integrator  InitialConditionSource=external  InitialCondition=45/57.3
  Integrator1 : Integrator
  Integrator2 : Integrator
  Product{,1..3,6} (5 alike) : Product
  Trigonometric Function : Trigonometry
  Trigonometric Function1 : Trigonometry  Operator=cos
  Trigonometric Function2 : Trigonometry  Operator=tan
  Trigonometric Function3 : Trigonometry  Operator=cos
  pitch : Outport
  psi : Outport  Port=2
  gamma : Outport  Port=3
  wires:
  Gain/1 -> Trigonometric Function3/1, Trigonometric Function2/1, pitch/1
  Divide/1 -> Integrator1/1
  Trigonometric Function1/1 -> Product2/2, Product1/2
  Add1/1 -> Product6/2, Divide/1
  Product3/1 -> Add1/2
  Integrator1/1 -> Gain1/1
  Integrator2/1 -> Gain2/1, Trigonometric Function1/1, Trigonometric Function/1
  omega_z/1 -> Product1/1, Product3/1
  Product2/1 -> Add1/1
  Trigonometric Function2/1 -> Product6/1
  Product/1 -> Add/1
  Trigonometric Function3/1 -> Divide/2
  Trigonometric Function/1 -> Product3/2, Product/2
  Product1/1 -> Add/2
  omega_y/1 -> Product/1, Product2/1
  Add/1 -> Integrator/1
  Add4/1 -> Integrator2/1
  omega_x/1 -> Add4/1
  Product6/1 -> Add4/2
  Constant/1 -> Integrator/2
  Integrator/1 -> Gain/1
  Gain1/1 -> psi/1
  Gain2/1 -> gamma/1
